simulink model "passivity1"  (Simulink 7.5)
settings: Solver=ode45  StartTime=0.0  StopTime=10.0  RelTol=1e-3
values from neighbouring files (symbols this model uses):
  alpha = 2    [pasivity1.m]
  am1 = 8    [pasivity1.m]
  am2 = 2    [pasivity1.m]
  bm1 = 2    [pasivity1.m]
  gama = 70    [pasivity1.m]
  p1 = P(1)    [pasivity1.m]
  p2 = P(2)    [pasivity1.m]
  r = 1    [pasivity1.m]
  T = 2*pi/10    (= 0.628318530718)    [pasivity1.m]
settings Model: Creator=mahtab  LastModifiedBy=morteza
settings DebuggingCC: FcnCallInpInsideContextMsg=Enable All
settings GRTTargetCC: CombineOutputUpdateFcns=on

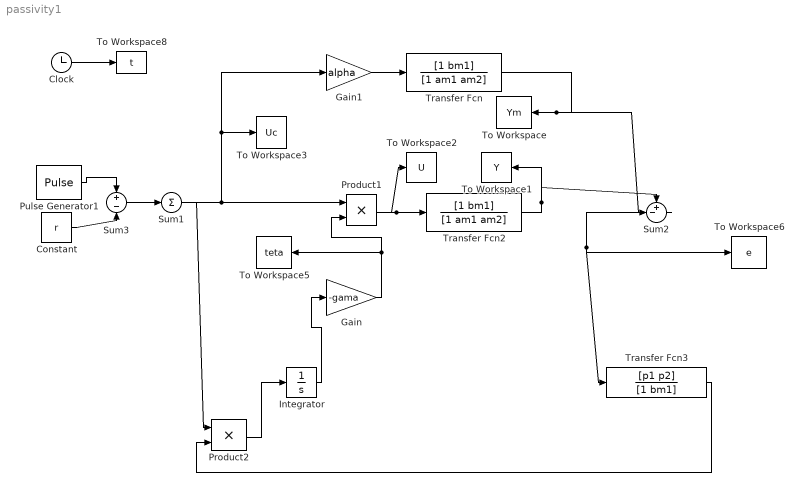
== system passivity1 ==
  Clock : Clock
      settings: Decimation=10
  Constant : Constant  Value=r
  Gain : Gain  Gain=-gama
  Gain1 : Gain  Gain=alpha
  Integrator : Integrator
  Product1 : Product  RndMeth=Zero
  Product2 : Product  RndMeth=Zero
  Pulse Generator1 : DiscretePulseGenerator  PulseType=Time based  Amplitude=2*r  Period=T  PulseWidth=50  PhaseDelay=0  SampleTime=1
  Sum1 : Sum  Inputs=+  SaturateOnIntegerOverflow=on
  Sum2 : Sum  Inputs=+-|  SaturateOnIntegerOverflow=on
  Sum3 : Sum  Inputs=+-  SaturateOnIntegerOverflow=on
  To Workspace : ToWorkspace  VariableName=Ym  SampleTime=-1  SaveFormat=Array
  To Workspace1 : ToWorkspace  VariableName=Y  SampleTime=-1  SaveFormat=Array
  To Workspace2 : ToWorkspace  VariableName=U  SampleTime=-1  SaveFormat=Array
  To Workspace3 : ToWorkspace  VariableName=Uc  SampleTime=-1  SaveFormat=Array
  To Workspace5 : ToWorkspace  VariableName=teta  SampleTime=-1  SaveFormat=Array
  To Workspace6 : ToWorkspace  VariableName=e  SampleTime=-1  SaveFormat=Array
  To Workspace8 : ToWorkspace  VariableName=t  SampleTime=-1  SaveFormat=Array
  Transfer Fcn : TransferFcn  Numerator=[1 bm1]  Denominator=[1 am1 am2]
  Transfer Fcn2 : TransferFcn  Numerator=[1 bm1]  Denominator=[1 am1 am2]
  Transfer Fcn3 : TransferFcn  Numerator=[p1 p2]  Denominator=[1 bm1]
  wires:
  Gain1/1 -> Transfer Fcn/1
  Product2/1 -> Integrator/1
  Pulse Generator1/1 -> Sum3/1
  Constant/1 -> Sum3/2
  Sum1/1 -> Product1/1, Gain1/1, To Workspace3/1, Product2/1
  Transfer Fcn3/1 -> Product2/2
  Sum2/1 -> Transfer Fcn3/1, To Workspace6/1
  Product1/1 -> Transfer Fcn2/1, To Workspace2/1
  Transfer Fcn2/1 -> To Workspace1/1, Sum2/1
  Clock/1 -> To Workspace8/1
  Transfer Fcn/1 -> To Workspace/1, Sum2/2
  Sum3/1 -> Sum1/1
  Integrator/1 -> Gain/1
  Gain/1 -> Product1/2, To Workspace5/1
